simulink library "csc_hvc_homography_velocity_covariance_lib"  (R2015b)
settings: Solver=VariableStepAuto  StartTime=0.0  StopTime=10.0  RelTol=1e-3
values from neighbouring files (symbols this model uses):
  mnc_meas_noise_alt = 8000.0    (= 8000)    [csc_mnc_measurement_noise_covariance_init.m]
  mnc_meas_noise_alt_gain = [0.2    0.2     1000   1000]    [csc_mnc_measurement_noise_covariance_init.m]
  mnc_R_lower_limit_alt = [0.0001 0.0001  10     10]    [csc_mnc_measurement_noise_covariance_init.m]
libraries: util_info_lib x1
settings Model: Creator=Mark Agbayani  LastModifiedBy=Mark Agbayani

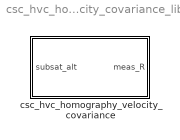
== system csc_hvc_homography_velocity_covariance_lib ==
  csc_hvc_homography_velocity_covariance : Subsystem

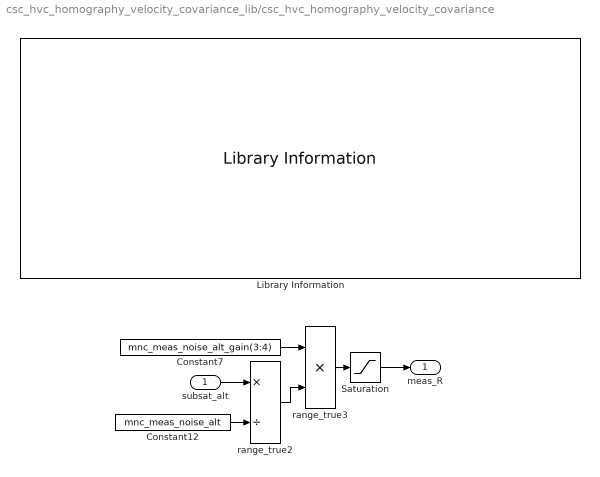
== system csc_hvc_homography_velocity_covariance_lib/csc_hvc_homography_velocity_covariance ==
  subsat_alt : Inport
  Constant12 : Constant  Value=mnc_meas_noise_alt
  Constant7 : Constant  Value=mnc_meas_noise_alt_gain(3:4)
  Library Information : util_info_lib/Library Information  owner='NONE'
  Saturation : Saturate  UpperLimit=1e20*[1 1]  LowerLimit=mnc_R_lower_limit_alt(3:4)
  range_true2 : Product  Inputs=*/  RndMeth=Zero
  range_true3 : Product  RndMeth=Zero
  meas_R : Outport
  wires:
  range_true2/1 -> range_true3/2
  Constant7/1 -> range_true3/1
  range_true3/1 -> Saturation/1
  Constant12/1 -> range_true2/2
  subsat_alt/1 -> range_true2/1
  Saturation/1 -> meas_R/1
